simulink model "impedanceControl2012b"  (Simulink 8.0)
settings: Solver=FixedStepDiscrete  StartTime=0.0  StopTime=simulationTime  FixedStep=Ts  RelTol=1e-3
InitFcn:
  | cd(fileparts(which(bdroot)));
  | init_impedanceControl;
values from neighbouring files (symbols this model uses):
  Kd = 0.0001    [init_impedanceControl.m]    (also in init_new_wbi_ID.m)
  Kp = 1/10*diag( ones(1,ROBOT_DOF)  )    [init_impedanceControl.m]    (also in init_new_wbi_ID.m = 1/2*diag( ones(1,ROBOT_DOF)  ))
  ROBOT_DOF = 2    [init.m]    (also in init_get_q.m = 1; init_impedanceControl.m = 23; init_new_wbi_ID.m = 3)
undefined symbols (not defined in the file or in its folder): AMPLS, FREQS, GRAV_COMP, MOVING
libraries: WBToolboxLibrary x13
settings Model: Creator=daniele  LastModifiedBy=DanielePucci
settings DataIOCC: SignalLoggingSaveFormat=ModelDataLogs
settings OptimizationCC: ExpressionDepthLimit=128
settings DebuggingCC: UnderspecifiedInitializationDetection=Simplified  MergeDetectMultiDrivingBlocksExec=error  MultiTaskDSMMsg=warning  MultiTaskCondExecSysMsg=none  FrameProcessingCompatibilityMsg=error  StateNameClashWarn=none  StrictBusMsg=ErrorOnBusTreatedAsVector
settings CodeAppCC: CustomSymbolStrType=$N$R$M_T
settings GRTTargetCC: CodeReplacementLibrary=C89/C90 (ANSI)

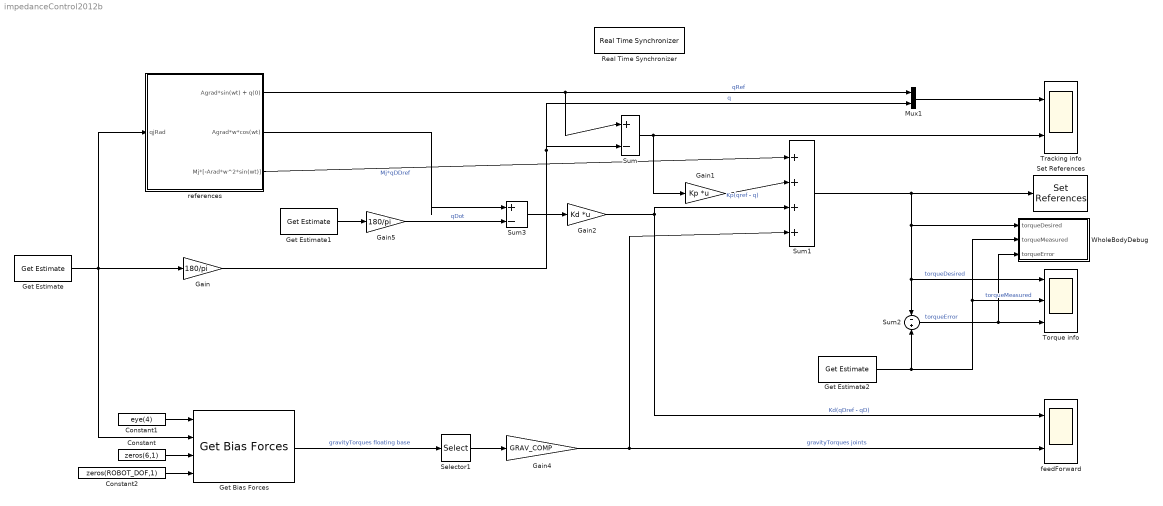
== system impedanceControl2012b ==
  Constant : Constant  Value=zeros(6,1)
  Constant1 : Constant  Value=eye(4)
  Constant2 : Constant  Value=zeros(ROBOT_DOF,1)
  Gain : Gain  Gain=180/pi
  Gain1 : Gain  Gain=Kp  Multiplication=Matrix(K*u)
  Gain2 : Gain  Gain=Kd  Multiplication=Matrix(K*u)
  Gain4 : Gain  Gain=GRAV_COMP
  Gain5 : Gain  Gain=180/pi
  Get Bias Forces : WBToolboxLibrary/wholeBodyModel/Dynamics/Get Bias Forces  robotName=WBT_robotName  localName=WBT_modelName  wbiFile=WBT_wbiFilename  wbiList=WBT_wbiList  explicitGravity=off
  Get Estimate : WBToolboxLibrary/wholeBodyStates/Get Estimate  estimateType=Joints Position  robotName=WBT_robotName  localName=WBT_modelName  wbiFile=WBT_wbiFilename  wbiList=WBT_wbiList
  Get Estimate1 : WBToolboxLibrary/wholeBodyStates/Get Estimate  estimateType=Joints Velocity  robotName=WBT_robotName  localName=WBT_modelName  wbiFile=WBT_wbiFilename  wbiList=WBT_wbiList
  Get Estimate2 : WBToolboxLibrary/wholeBodyStates/Get Estimate  estimateType=Joints Torque  robotName=WBT_robotName  localName=WBT_modelName  wbiFile=WBT_wbiFilename  wbiList=WBT_wbiList
  Mux1 : Mux  Inputs=2
  Real Time Synchronizer : WBToolboxLibrary/Utilities/Real Time Synchronizer  period=0.01
  Selector1 : Selector  InputPortWidth=ROBOT_DOF+6  IndexOptions=Index vector (dialog)  Indices=[7:ROBOT_DOF+6]  OutputSizes=1
  Set References : WBToolboxLibrary/wholeBodyActuators/Set References  controlType=Torque  robotName=WBT_robotName  localName=WBT_modelName  wbiFile=WBT_wbiFilename  wbiList=WBT_wbiList
  Sum : Sum  Inputs=|+-
  Sum1 : Sum  Inputs=|++++
  Sum2 : Sum  Inputs=-|+
  Sum3 : Sum  Inputs=|+-
  Torque info : Scope  NumInputPorts=3
      settings: TimeRange=20  ShowLegends=on  MaxDataPoints=5000  SaveToWorkspace=off  SaveName=ScopeData  YMin=-3~-2~-2  YMax=3~3~2  SampleTime=-1  DataFormat=Array
  Tracking info : Scope  NumInputPorts=2
      settings: TimeRange=20  ShowLegends=on  MaxDataPoints=5000  SaveToWorkspace=off  SaveName=ScopeData3  YMin=-65.50412~-21.92946  YMax=79.53709~20.97556  SampleTime=-1  DataFormat=Array
  WholeBodyDebug : Subsystem
  feedForward : Scope  NumInputPorts=2
      settings: TimeRange=70  ShowLegends=on  MaxDataPoints=5000  SaveToWorkspace=off  YMin=-5~-5  YMax=4~5  SampleTime=-1  DataFormat=Array
  references : Subsystem
  wires:
  Gain/1 -> Mux1/2, Sum/2  "q"
  Sum/1 -> Gain1/1, Tracking info/2
  Gain1/1 -> Sum1/2  "Kp(qref - q)"
  Gain2/1 -> feedForward/1, Sum1/3  "Kd(qDref - qD)"
  Sum1/1 -> Set References/1, Sum2/1, Torque info/1, WholeBodyDebug/1(torqueDesired)  "torqueDesired"
  Constant/1 -> Get Bias Forces/3
  Get Bias Forces/1 -> Selector1/1  "gravityTorques floating base"
  Get Estimate/1 -> Gain/1, references/1(qjRad), Get Bias Forces/2
  Selector1/1 -> Gain4/1
  Get Estimate2/1 -> WholeBodyDebug/2(torqueMeasured), Torque info/2, Sum2/2  "torqueMeasured"
  Sum2/1 -> WholeBodyDebug/3(torqueError), Torque info/3  "torqueError"
  Mux1/1 -> Tracking info/1
  references/1(Agrad*sin(wt) + q(0)) -> Mux1/1, Sum/1  "qRef"
  Gain5/1 -> Sum3/2  "qDot"
  Sum3/1 -> Gain2/1
  references/2(Agrad*w*cos(wt)) -> Sum3/1
  references/3(Mj*[-Arad*w^2*sin(wt)]) -> Sum1/1  "Mj*qDDref"
  Constant1/1 -> Get Bias Forces/1
  Gain4/1 -> Sum1/4, feedForward/2  "gravityTorques joints"
  Get Estimate1/1 -> Gain5/1
  Constant2/1 -> Get Bias Forces/4

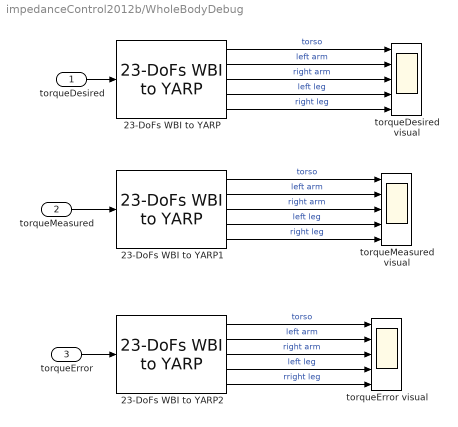
== system impedanceControl2012b/WholeBodyDebug ==
  torqueDesired : Inport
  torqueMeasured : Inport  Port=2
  torqueError : Inport  Port=3
  23-DoFs WBI to YARP : WBToolboxLibrary/Utilities/23-DoFs WBI to YARP
  23-DoFs WBI to YARP1 : WBToolboxLibrary/Utilities/23-DoFs WBI to YARP
  23-DoFs WBI to YARP2 : WBToolboxLibrary/Utilities/23-DoFs WBI to YARP
  torqueDesired visual : Scope  NumInputPorts=5
      settings: TimeRange=auto  MaxDataPoints=5000  SaveToWorkspace=off  SaveName=ScopeData4  YMin=-10.60669~-4.41981~-4.32368~-9.75297~-9.79728  YMax=8.23515~3.13837~3.20996~11.78733~12.0506  SampleTime=-1
  torqueError visual : Scope  NumInputPorts=5
      settings: TimeRange=auto  MaxDataPoints=5000  SaveToWorkspace=off  SaveName=ScopeData6  YMin=-8.62947~-2.17391~-1.9799~-9.84767~-9.99343  YMax=10.37752~2.14997~2.02026~10.72787~9.36263  SampleTime=-1
  torqueMeasured visual : Scope  NumInputPorts=5
      settings: TimeRange=auto  MaxDataPoints=5000  SaveToWorkspace=off  SaveName=ScopeData5  YMin=-3.9166~-2.90657~-3.40764~-3.91105~-4.23065  YMax=0.8634~1.91659~2.31467~7.95355~8.01662  SampleTime=-1
  wires:
  torqueMeasured/1 -> 23-DoFs WBI to YARP1/1
  torqueError/1 -> 23-DoFs WBI to YARP2/1
  torqueDesired/1 -> 23-DoFs WBI to YARP/1
  23-DoFs WBI to YARP/1 -> torqueDesired visual/1  "torso"
  23-DoFs WBI to YARP/2 -> torqueDesired visual/2  "left arm"
  23-DoFs WBI to YARP/3 -> torqueDesired visual/3  "right arm"
  23-DoFs WBI to YARP/4 -> torqueDesired visual/4  "left leg"
  23-DoFs WBI to YARP/5 -> torqueDesired visual/5  "right leg"
  23-DoFs WBI to YARP1/1 -> torqueMeasured visual/1  "torso"
  23-DoFs WBI to YARP1/2 -> torqueMeasured visual/2  "left arm"
  23-DoFs WBI to YARP1/3 -> torqueMeasured visual/3  "right arm"
  23-DoFs WBI to YARP1/4 -> torqueMeasured visual/4  "left leg"
  23-DoFs WBI to YARP1/5 -> torqueMeasured visual/5  "right leg"
  23-DoFs WBI to YARP2/1 -> torqueError visual/1  "torso"
  23-DoFs WBI to YARP2/2 -> torqueError visual/2  "left arm"
  23-DoFs WBI to YARP2/3 -> torqueError visual/3  "right arm"
  23-DoFs WBI to YARP2/4 -> torqueError visual/4  "left leg"
  23-DoFs WBI to YARP2/5 -> torqueError visual/5  "rright leg"

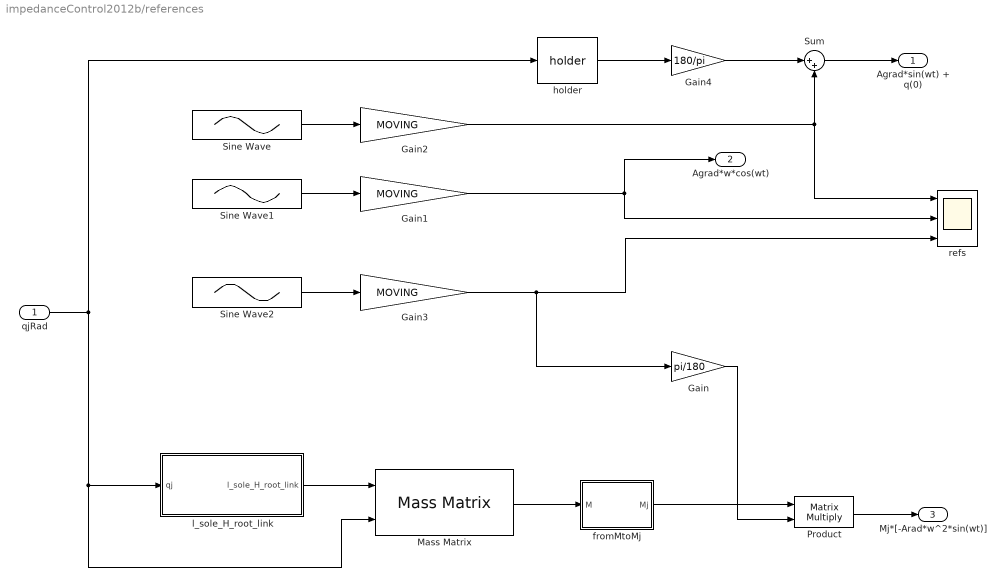
== system impedanceControl2012b/references ==
  qjRad : Inport
  Gain : Gain  Gain=pi/180
  Gain1 : Gain  Gain=MOVING
  Gain2 : Gain  Gain=MOVING
  Gain3 : Gain  Gain=MOVING
  Gain4 : Gain  Gain=180/pi
  Mass Matrix : WBToolboxLibrary/wholeBodyModel/Dynamics/Mass Matrix  robotName=WBT_robotName  localName=WBT_modelName  wbiFile=WBT_wbiFilename  wbiList=WBT_wbiList
  Product : Product  Multiplication=Matrix(*)
  Sine Wave : Sin  Amplitude=AMPLS  Frequency=FREQS*2*pi  SampleTime=0
  Sine Wave1 : Sin  Amplitude=AMPLS.*FREQS*2*pi  Frequency=FREQS*2*pi  Phase=pi/2  SampleTime=0
  Sine Wave2 : Sin  Amplitude=-AMPLS.*(FREQS*2*pi).^2  Frequency=FREQS*2*pi  SampleTime=0
  Sum : Sum  Inputs=|++
  fromMtoMj : MATLAB Function  TreatAsAtomicUnit=on
      settings: PermitHierarchicalResolution=ParametersOnly
  "holder " : WBToolboxLibrary/Utilities/holder 
  l_sole_H_root_link : Subsystem
  refs : Scope  NumInputPorts=3
      settings: TimeRange=70  ShowLegends=on  MaxDataPoints=5000  SaveToWorkspace=off  SaveName=ScopeData2  YMin=-5~-5~-5  YMax=4~5~5  SampleTime=-1  DataFormat=Array
  Agrad*sin(wt) + q(0) : Outport
  Agrad*w*cos(wt) : Outport  Port=2
  Mj*[-Arad*w^2*sin(wt)] : Outport  Port=3
  wires:
  Sine Wave/1 -> Gain2/1
  Gain2/1 -> Sum/2, refs/1
  Sine Wave1/1 -> Gain1/1
  Gain1/1 -> refs/2, Agrad*w*cos(wt)/1
  Sine Wave2/1 -> Gain3/1
  Product/1 -> Mj*[-Arad*w^2*sin(wt)]/1
  Mass Matrix/1 -> fromMtoMj/1(M)
  fromMtoMj/1(Mj) -> Product/1
  Gain3/1 -> refs/3, Gain/1
  Gain/1 -> Product/2
  qjRad/1 -> "holder "/1, l_sole_H_root_link/1(qj), Mass Matrix/2
  Sum/1 -> Agrad*sin(wt) + q(0)/1
  "holder "/1 -> Gain4/1
  Gain4/1 -> Sum/1
  l_sole_H_root_link/1(l_sole_H_root_link) -> Mass Matrix/1

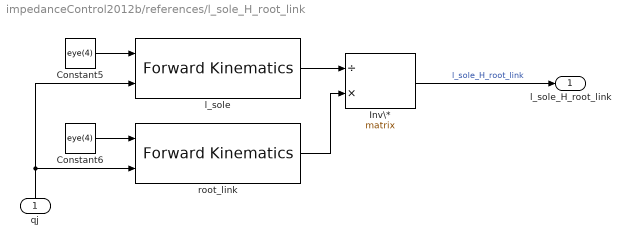
== system impedanceControl2012b/references/l_sole_H_root_link ==
  qj : Inport
  Constant5 : Constant  Value=eye(4)
  Constant6 : Constant  Value=eye(4)
  Inv\* : Product  Inputs=/*  Multiplication=Matrix(*)
  l_sole : WBToolboxLibrary/wholeBodyModel/Kinematics/Forward Kinematics  frameName='l_sole'  robotName=WBT_robotName  localName=WBT_modelName  wbiFile=WBT_wbiFilename  wbiList=WBT_wbiList
  root_link : WBToolboxLibrary/wholeBodyModel/Kinematics/Forward Kinematics  frameName='root_link'  robotName=WBT_robotName  localName=WBT_modelName  wbiFile=WBT_wbiFilename  wbiList=WBT_wbiList
  l_sole_H_root_link : Outport
  wires:
  Constant5/1 -> l_sole/1
  Inv\*/1 -> l_sole_H_root_link/1  "l_sole_H_root_link"
  l_sole/1 -> Inv\*/1
  Constant6/1 -> root_link/1
  qj/1 -> l_sole/2, root_link/2
  root_link/1 -> Inv\*/2

== matlab function references/fromMtoMj ==
  data: M input double; Mj output double
function Mj = fromMtoMj(M)
%#codegen

Mj = M(7:end,7:end);
